simulink model "UpperLimb_Optimization"  (R2024b)
settings: Solver=VariableStepAuto  StartTime=0.0  StopTime=10.0  RelTol=1e-3
settings Model: Creator=jakub  LastModifiedBy=jakub

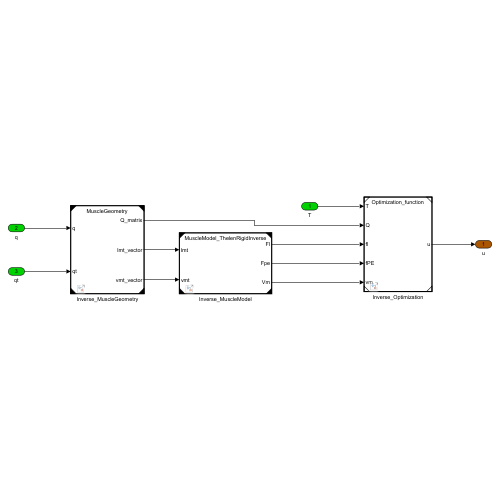
[thumbnail: Simulink's stored preview of the top-level diagram]
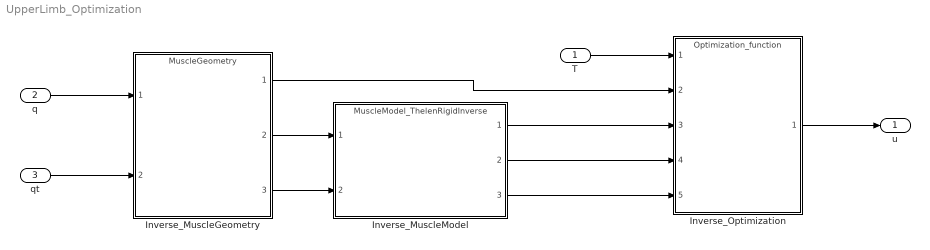
== system UpperLimb_Optimization ==
  T : Inport  OutDataTypeStr=double  Unit=N*m  PortDimensions=[2 1]  SampleTime=0
  q : Inport  Port=2  OutDataTypeStr=double  Unit=rad  PortDimensions=[2 1]  SampleTime=0
  qt : Inport  Port=3  OutDataTypeStr=double  Unit=rad/sec  PortDimensions=[2 1]  SampleTime=0
  Inverse_MuscleGeometry : ModelReference  ModelNameDialog=MuscleGeometry.slx  ModelReferenceVersion=1.153
  Inverse_MuscleModel : ModelReference  ModelNameDialog=MuscleModel_ThelenRigidInverse.slx  ModelReferenceVersion=1.21
  Inverse_Optimization : ModelReference  ModelNameDialog=Optimization_function.slx  SimulationMode=Normal  ModelReferenceVersion=1.11
  u : Outport  OutDataTypeStr=double  PortDimensions=[8 1]  SampleTime=0
  wires:
  Inverse_MuscleModel/3 -> Inverse_Optimization/5
  Inverse_MuscleModel/2 -> Inverse_Optimization/4
  Inverse_MuscleModel/1 -> Inverse_Optimization/3
  T/1 -> Inverse_Optimization/1
  Inverse_Optimization/1 -> u/1
  Inverse_MuscleGeometry/3 -> Inverse_MuscleModel/2
  Inverse_MuscleGeometry/2 -> Inverse_MuscleModel/1
  qt/1 -> Inverse_MuscleGeometry/2
  q/1 -> Inverse_MuscleGeometry/1
  Inverse_MuscleGeometry/1 -> Inverse_Optimization/2
